simulink model "sl_lanechange"  (Simulink 8.3)
settings: Solver=ode45  StartTime=0.0  StopTime=10.0  RelTol=1e-3
libraries: simulink x2, roblocks x1
settings Model: Creator=pic  LastModifiedBy=Administrator
settings OptimizationCC: ExpressionDepthLimit=2147483647
settings DebuggingCC: FcnCallInpInsideContextMsg=UseLocalSettings

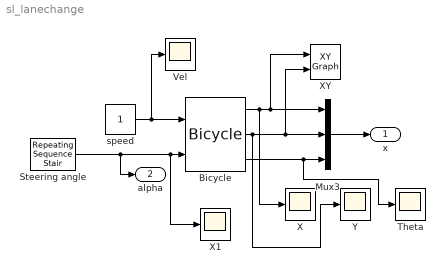
== system sl_lanechange ==
  Bicycle : roblocks/Dynamics/Bicycle  accel=1  vlim=1  alim=2  L=1  x0=[0, 0, 0]  handbrake=0
  Mux3 : Mux  Inputs=3
  Steering angle : simulink/Sources/Repeating Sequence Stair  OutValues=[0 0 0 1 0 -1 0 0 0 0]  tsamp=1  OutMin=[]  OutMax=[]  OutDataTypeStr=double  OutputDataTypeScalingMode=Specify via dialog  OutDataType=double  ConRadixGroup=Best Precision: Vector-wise  OutScaling=2^-12
  Theta : Scope
      settings: SaveName=ScopeData4
  Vel : Scope
  X : Scope
  X1 : Scope
      settings: SaveName=ScopeData3
  XY : simulink/Sinks/XY Graph  xmin=0  xmax=10  ymin=0  ymax=5  st=-1
  Y : Scope
      settings: SaveName=ScopeData2
  speed : Constant  VectorParams1D=off  SampleTime=0.02
  x : Outport
  alpha : Outport  Port=2
  wires:
  Steering angle/1 -> alpha/1, X1/1, Bicycle/2
  speed/1 -> Vel/1, Bicycle/1
  Bicycle/3 -> Theta/1, Mux3/3
  Bicycle/1 -> X/1, Mux3/1, XY/1
  Bicycle/2 -> Y/1, Mux3/2, XY/2
  Mux3/1 -> x/1
